simulink model "robot_state_machine"  (R2018b)
settings: Solver=FixedStepDiscrete  StartTime=0.0  StopTime=10.0  FixedStep=0.1  RelTol=1e-3  EnableMultiTasking=on
settings Model: Creator=larry  LastModifiedBy=larry
settings SolverCC: AutoInsertRateTranBlk=on
settings DataIOCC: LimitDataPoints=on
settings OptimizationCC: LifeSpan=inf
settings DebuggingCC: AllowSymbolicDim=off  SFUnexpectedBacktrackingDiag=warning  SFNoUnconditionalDefaultTransitionDiag=warning  SFExecutionAtInitializationDiag=none
settings SFSimCC: SimUseLocalCustomCode=off
settings RTWCC: RTWUseLocalCustomCode=off
settings CodeAppCC: StateflowObjectComments=on
settings GRTTargetCC: TargetLangStandard=C89/C90 (ANSI)
settings ConfigComp: CovMetricSettings=dw  CovHtmlReporting=on  CovSaveCumulativeToWorkspaceVar=on  CovSaveSingleToWorkspaceVar=on  CovShowResultsExplorer=off  CovExternalEMLEnable=off

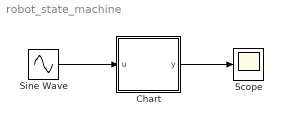
== system robot_state_machine ==
  Chart : Stateflow chart  TreatAsAtomicUnit=on
  Scope : Scope
  Sine Wave : Sin  SampleTime=0
  wires:
  Sine Wave/1 -> Chart/1(u)
  Chart/1(y) -> Scope/1

== stateflow chart robot_state_machine/Chart ==
  state DISABLED
    entry: y = -1; % entry action
    % during:
  state AUTONOMOUS_ENABLED
    entry: y = 1;
  note: Robot Mode
  state TELEOPERATED_ENABLED
    entry: y = 1;
  state VISION_DISABLED
  state VISION_STREAM
  state VISION_START_UP
  note: Vision
  state VISION_HATCH
  state DRIVE_DISABLED
  state MANUAL_DRIVE
  state VISION_READY
  state VISION_TARGET
  state DRIVE_READY
    % check hardware
  state GUIDED_ALIGNMENT
  note: Drive
  state VISION_LINE
  state PATH_FOLLOWING
  state RAMP_FOLDED
  state RAMP_DEPLOYED
  note: Ramp
  state RAMP_READY
    % check hardware?
  state RAMP_PARTIALLY_RETRACTED
  (default) -> DISABLED [order 1]
  DISABLED -> AUTONOMOUS_ENABLED [order 1] : [u <= 0]
      | % [transition condition]{action}
  AUTONOMOUS_ENABLED -> DISABLED : [u > 0]
  TELEOPERATED_ENABLED -> DISABLED
  DISABLED -> TELEOPERATED_ENABLED [order 2]
  (default) -> VISION_DISABLED [order 4]
  VISION_READY -> VISION_DISABLED [order 1]
  VISION_DISABLED -> VISION_START_UP
  VISION_READY -> VISION_STREAM [order 3]
  VISION_STREAM -> VISION_READY
  (default) -> DRIVE_DISABLED [order 2]
  VISION_START_UP -> VISION_READY
  VISION_HATCH -> VISION_READY
  VISION_READY -> VISION_HATCH [order 2]
  MANUAL_DRIVE -> DRIVE_DISABLED [order 1]
  PATH_FOLLOWING -> MANUAL_DRIVE [order 2] : % finished
  DRIVE_READY -> MANUAL_DRIVE [order 2]
  GUIDED_ALIGNMENT -> DRIVE_DISABLED [order 1]
  MANUAL_DRIVE -> DRIVE_READY [order 2]
  PATH_FOLLOWING -> DRIVE_DISABLED [order 1]
  VISION_LINE -> VISION_READY
  VISION_READY -> VISION_LINE [order 5]
  VISION_TARGET -> VISION_READY
  VISION_READY -> VISION_TARGET [order 4]
  GUIDED_ALIGNMENT -> MANUAL_DRIVE [order 2] : % finished
  DRIVE_READY -> DRIVE_DISABLED [order 1]
  DRIVE_DISABLED -> DRIVE_READY
  DRIVE_READY -> GUIDED_ALIGNMENT [order 3]
  DRIVE_READY -> PATH_FOLLOWING [order 4]
  (default) -> RAMP_FOLDED [order 3]
  RAMP_READY -> RAMP_DEPLOYED [order 2]
  RAMP_DEPLOYED -> RAMP_PARTIALLY_RETRACTED
  RAMP_READY -> RAMP_FOLDED [order 1]
  RAMP_FOLDED -> RAMP_READY
  data: u input; y output
